simulink model "pendulum_rwp_v2"  (R2022a)
settings: Solver=VariableStepAuto  StartTime=0.0  StopTime=10  MaxStep=0.01  RelTol=1e-3  EnableMultiTasking=on
values from neighbouring files (symbols this model uses):
  a = m1*l1^2 + m1*l2^2 + J1 + J2    (= 0.01390808)    [simulate_the_effect_of_inertia_moment_j2.m]
  b = m1*l1 + m2*l2    (= 0.07644)    [simulate_the_effect_of_inertia_moment_j2.m]
  c1 = 0.004    [simulate_the_effect_of_inertia_moment_j2.m]
  c2 = 0.0007    [simulate_the_effect_of_inertia_moment_j2.m]
  dcm_on = 0    [simulate_the_effect_of_inertia_moment_j2.m]
  g = 9.81    [simulate_the_effect_of_inertia_moment_j2.m]
  J2 = 0.00001    (= 1e-05)    [simulate_the_effect_of_inertia_moment_j2.m]
  Kb = 0.0987    [simulate_the_effect_of_inertia_moment_j2.m]
  Kt = 0.0987    [simulate_the_effect_of_inertia_moment_j2.m]
  Ra = 32.6    [simulate_the_effect_of_inertia_moment_j2.m]
  theta_0 = 14.94*pi/180 + pi    (= 3.40234484384)    [simulate_the_effect_of_inertia_moment_j2.m]
  Vm = 12    [simulate_the_effect_of_inertia_moment_j2.m]
libraries: simulink_extras x1
Description:
  | modified 22.10.2021
settings Model: Creator=TL RT-Lab  LastModifiedBy=adlipke
settings Model: ModifiedHistory=|
  | init: Okt. 2021
  | current version v2
settings SolverCC: AlgebraicLoopSolver=TrustRegion
settings DataIOCC: SaveFormat=Array  SaveOutput=off  SignalLogging=off  DSMLogging=off  SaveTime=off  ReturnWorkspaceOutputs=off
settings OptimizationCC: OptimizeBlockIOStorage=off  BufferReuse=off  GlobalBufferReuse=off  ExpressionFolding=off  LocalBlockOutputs=off  LifeSpan=inf
settings DebuggingCC: SolverPrmCheckMsg=warning  UnconnectedInputMsg=warning  UnconnectedOutputMsg=warning  UnconnectedLineMsg=warning  AllowSymbolicDim=off  SFUnexpectedBacktrackingDiag=warning  SFNoUnconditionalDefaultTransitionDiag=warning  SFExecutionAtInitializationDiag=none  SFMachineParentedDataDiag=warning  ArithmeticOperatorsInVariantConditions=warning
settings HardwareCC: ProdBitPerPointer=32  ProdBitPerSizeT=32  ProdBitPerPtrDiffT=32  ProdLargestAtomicFloat=None  ProdIntDivRoundTo=Undefined  ProdEndianess=Unspecified  ProdWordSize=32  ProdHWDeviceType=32-bit Generic
settings ModelReferenceCC: PropagateSignalLabelsOutOfModel=off
settings SFSimCC: SimUseLocalCustomCode=off  CustomCodeUndefinedFunction=UseInterfaceOnly
settings RTWCC: RTWUseLocalCustomCode=off  DLArmComputeVersion=19.05
settings CodeAppCC: StateflowObjectComments=on
settings GRTTargetCC: TargetLangStandard=C89/C90 (ANSI)
settings ConfigComp: CovMetricSettings=dw  CovSaveCumulativeToWorkspaceVar=on  CovSaveSingleToWorkspaceVar=on  CovExternalEMLEnable=off

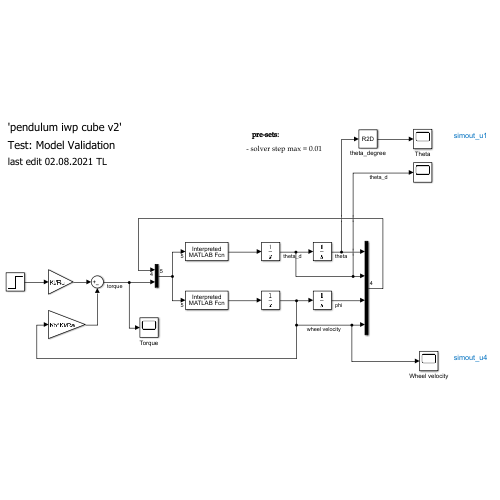
[thumbnail: Simulink's stored preview of the top-level diagram]
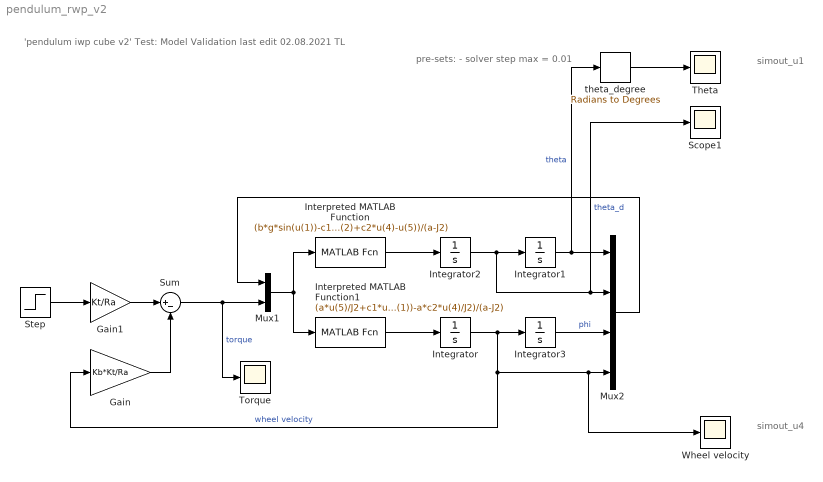
== system pendulum_rwp_v2 ==
  note: 'pendulum iwp cube v2'
      |
      | Test: Model Validation
      |
      | last edit 02.08.2021 TL
  note: pre-sets:
      |
      | - solver step max = 0.01
  note: simout_u1
  note: simout_u4
  Gain : Gain  Gain=Kb*Kt/Ra
  Gain1 : Gain  Gain=Kt/Ra
  Integrator : Integrator
  Integrator1 : Integrator  InitialCondition=theta_0
  Integrator2 : Integrator
  Integrator3 : Integrator
  Interpreted MATLAB Function : MATLABFcn  MATLABFcn=(b*g*sin(u(1))-c1*u(2)+c2*u(4)-u(5))/(a-J2)  Output1D=off
  Interpreted MATLAB Function1 : MATLABFcn  MATLABFcn=(a*u(5)/J2+c1*u(2)-b*g*sin(u(1))-a*c2*u(4)/J2)/(a-J2)  Output1D=off
  Mux1 : Mux  Inputs=2
  Mux2 : Mux
  Scope1 : Scope
  Step : Step  Time=dcm_on  After=Vm  SampleTime=0
  Sum : Sum  Inputs=|+-
  Theta : Scope
  Torque : Scope
  Wheel velocity : Scope
  theta_degree : simulink_extras/Transformations/Radians to Degrees
  wires:
  Interpreted MATLAB Function/1 -> Integrator2/1
  Integrator2/1 -> Integrator1/1, Scope1/1, Mux2/2  "theta_d"
  Integrator1/1 -> theta_degree/1, Mux2/1  "theta"
  Integrator3/1 -> Mux2/3  "phi"
  Interpreted MATLAB Function1/1 -> Integrator/1
  Mux1/1 -> Interpreted MATLAB Function1/1, Interpreted MATLAB Function/1
  Mux2/1 -> Mux1/1
  Sum/1 -> Torque/1, Mux1/2  "torque"
  Gain/1 -> Sum/2
  Integrator/1 -> Wheel velocity/1, Mux2/4, Gain/1, Integrator3/1  "wheel velocity"
  Gain1/1 -> Sum/1
  theta_degree/1 -> Theta/1
  Step/1 -> Gain1/1
